simulink model "IEEE_39bus_load_increase_vol1"  (R2024b)
settings: Solver=ode23tb  StartTime=0.0  StopTime=500  MaxStep=1/60  RelTol=1e-2  AbsTol=1e-1  EnableMultiTasking=on
PreLoadFcn:
  | NE39bus_data;
  | PSSMODEL=1;
  | LPSS=0;
  | WAPSS=0;
  | WAPSS2=0;
values from neighbouring files (symbols this model uses):
  deg = [19.62;0;2.466;4.423;3.398;5.698;8.494;2.181;7.784;-3.646]*pi/180    [main_39.m]
  ki_sapc = 0.02*2.5/4    (= 0.0125)    [main_39.m]
  kp = 5*ones(10,1)    [main_39.m]
  kp_sapc = 0.15*1.25    (= 0.1875)    [main_39.m]
  line = [     1	2	0.0035	0.0411	0.6987	0	100	345 ... (first row only)    [main_39.m]
  P_base = mac_con(:,3).*[0.5609;0.6011;0.6995;0.6432;0.5143;0.6634;0.5676;0.5897;0.8444;0.3464]    [main_39.m]
  P_cmd = [1.140 	1.060 	1.100 	1.120 	0	1.060 	1.115 	1.160 	1.175 	1.000 ]    [main_39.m]
  Pmax = [1.20; 1.10; 1.15; 1.15;1.10;1.10;1.15;1.20;1.20;1.00]    [main_39.m]
  Pmin = 2-Pmax    [main_39.m]
  s = 10    [main_39.m]
  ts_pi = 5    [main_39.m]
  Udc = 2*Bus(mac_con(:,2),2)*1e3    [main_39.m]
  V_m = [1.03;0.982;0.9831;0.9972;1.0123;1.0493;1.0635;1.0278;1.0265;1.048]*sqrt(2/3)    [main_39.m]
undefined symbols (not defined in the file or in its folder): D1, Delta
libraries: spsThreePhaseVIMeasurementLib x40, spsThreePhasePISectionLineLib x34, spsThreePhaseParallelRLCLoadLib x21, spsThreePhaseTransformerTwoWindingsLib x13, spsMeanLib x12, slpidlib x12, spsLoadFlowBusLib x10, spsPLL3phLib x10, spsPowerPositiveSequenceLib x10, spsDCVoltageSourceLib x10, simulink x10, spsUniversalBridgeLib x10
(part 3 of 4)

== system IEEE_39bus_load_increase_vol1/VSC3/sapc ==
  In1 : Inport
  In2 : Inport  Port=2
  Abs1 : Abs  SaturateOnIntegerOverflow=off
  Constant : Constant  Value=kp_sapc
  Constant1 : Constant  Value=ki_sapc
  Constant2 : Constant  Value=1/0.015
  Constant3 : Constant  Value=1.5
  Constant4 : Constant  Value=0.016
  Delay : Delay  DelayLength=1  InitialCondition=0  SampleTime=1e-4
  Delay1 : Delay  DelayLength=1  InitialCondition=0  SampleTime=1e-4
  Delay2 : Delay  DelayLength=1  InitialCondition=0  SampleTime=1e-4
  Discrete PID Controller : slpidlib/PID Controller  Controller=PI  Form=Parallel  TimeDomain=Discrete-time  UseExternalTs=off  SampleTime=-1  IntegratorMethod=Forward Euler  FilterMethod=Forward Euler  ControllerParametersSource=external  P=kp_sapc  I=ki_sapc  UseKiTs=off  D=0  UseExternalDerivativeSource=off  N=100  UseFilter=on  TunerSelectOption=Transfer Function Based (PID Tuner App)  InitialConditionSource=internal  InitialConditionForIntegrator=0  InitialConditionForFilter=0  DifferentiatorICPrevScaledInput=0  ExternalReset=none  TrackingMode=off  Kt=1  LimitOutput=off  SatLimitsSource=internal  UpperSaturationLimit=inf  LowerSaturationLimit=-inf  LinearizeAsGain=off  AntiWindupMode=none  Kb=1  LimitIntegrator=off  UpperIntegratorSaturationLimit=inf  LowerIntegratorSaturationLimit=-inf  POutMin=[]  POutMax=[]  IOutMin=[]  IOutMax=[]  DOutMin=[]  DOutMax=[]  NOutMin=[]  NOutMax=[]  SumOutMin=[]  SumOutMax=[]  SaturationOutMin=[]  SaturationOutMax=[]  PParamMin=[]  PParamMax=[]  IParamMin=[]  IParamMax=[]  DParamMin=[]  DParamMax=[]  NParamMin=[]  NParamMax=[]  KbParamMin=[]  KbParamMax=[]  KtParamMin=[]  KtParamMax=[]  KbOutMin=[]  KbOutMax=[]  KtOutMin=[]  KtOutMax=[]  IntegratorOutMin=[]  IntegratorOutMax=[]  FilterOutMin=[]  FilterOutMax=[]  SumI1OutMin=[]  SumI1OutMax=[]  SumI2OutMin=[]  SumI2OutMax=[]  SumI3OutMin=[]  SumI3OutMax=[]  SumI4OutMin=[]  SumI4OutMax=[]  SumDOutMin=[]  SumDOutMax=[]  DifferentiatorOutMin=[]  DifferentiatorOutMax=[]  FilterDiffOutCoefMin=[]  FilterDiffOutCoefMax=[]  ReciprocalOutMin=[]  ReciprocalOutMax=[]  SumDenOutMin=[]  SumDenOutMax=[]  SumNumOutMin=[]  SumNumOutMax=[]  DivideOutMin=[]  DivideOutMax=[]  UdiffTsProdOutMin=[]  UdiffTsProdOutMax=[]  NTsProdOutMin=[]  NTsProdOutMax=[]  UintegralTsProdOutMin=[]  UintegralTsProdOutMax=[]  UngainTsProdOutMin=[]  UngainTsProdOutMax=[]  ClampingZeroOutDataTypeStr=Inherit: Inherit via back propagation  ClampingZeroOutMin=[]  ClampingZeroOutMax=[]  FilterDenConstantOutDataTypeStr=Inherit: Inherit via back propagation  FilterDenConstantOutMin=[]  FilterDenConstantOutMax=[]  PCopyOutDataTypeStr=Inherit: Inherit via back propagation  PCopyOutMin=[]  PCopyOutMax=[]  NCopyOutDataTypeStr=Inherit: Inherit via back propagation  NCopyOutMin=[]  NCopyOutMax=[]  IntegratorContinuousStateAttributes=''  IntegratorStateMustResolveToSignalObject=off  IntegratorRTWStateStorageClass=Auto  FilterContinuousStateAttributes=''  FilterStateMustResolveToSignalObject=off  FilterRTWStateStorageClass=Auto  ParallelPVariant=ExternalParameters  IdealPVariant=Disabled  IVariant=ExternalParameters  DVariant=Disabled  IntegratorVariant=Discrete  SatVariant=Disabled  AWVariant=Passthrough  PCopyVariant=Disabled  TRVariant=Disabled  FdbkBlocksVariant=Forward  IdealPFdbkVariant=Disabled  SatFdbkVariant=Disabled  DerivativeFilterVariant=Disabled  NVariant=Disabled  NCopyVariant=Disabled_SignalSpec  FilterICVariant=Disabled  IntegratorICVariant=InternalICs  ExternalResetVariant=Disabled  TRSumVariant=Passthrough  SumFdbkVariant=Disabled  SumVariant=Sum_PI  TsampFilterVariant=InternalTs  TsampNgainVariant=Passthrough  TsampIntegralVariant=Disabled_SignalSpec  ExternalSaturationOutDataTypeStr=Inherit: Same as second input  DerivativeSourceVariant=Disabled  PreIntVariant=InternalPreInt
      settings: LibrarySourceBlock=simulink/Discrete/Discrete PID Controller
  Gain1 : Gain  Gain=1/0.015/0.015
  Gain2 : Gain  Gain=1/2
  Gain4 : Gain  Gain=P_base(3)/1e3
  Product{,1..5} (6 alike) : Product
  Saturation : Saturate  UpperLimit=1  LowerLimit=1
  Saturation1 : Saturate  UpperLimit=1  LowerLimit=0
  Scope1 : Scope  NumInputPorts=3
  Scope2 : Scope  NumInputPorts=2
  Step : Step  Time=15  SampleTime=0
  Sum : Sum  Inputs=|+-
  Sum1 : Sum  Inputs=|+-
  Sum2 : Sum  Inputs=|+-
  Sum3 : Sum  Inputs=|++
  Zero-Order Hold : ZeroOrderHold  SampleTime=ts_pi
  delta : Outport
  tag scope: delta_sapc3=global
  wires:
  Product/1 -> [delta_sapc3], Scope1/3, Discrete PID Controller/1
  Step/1 -> Product/2
  Sum/1 -> Gain4/1
  Discrete PID Controller/1 -> Scope1/1, Zero-Order Hold/1
  In1/1 -> Sum/1
  In2/1 -> Sum/2
  Zero-Order Hold/1 -> Scope1/2, Delay1/1
  Product2/1 -> Scope2/2, Discrete PID Controller/3
  Constant/1 -> Product1/1
  Saturation/1 -> Product2/1, Product1/2
  Product1/1 -> Scope2/1, Discrete PID Controller/2
  Constant1/1 -> Product2/2
  Constant4/1 -> Sum1/1
  Abs1/1 -> Product5/2, Sum1/2
  Constant3/1 -> Sum2/1
  Product3/1 -> Gain1/1
  Gain1/1 -> Delay/1
  Sum1/1 -> Product3/1, Product3/2
  Gain4/1 -> Abs1/1, Product/1
  Delay/1 -> Sum2/2
  Delay1/1 -> delta/1
  Product5/1 -> Saturation1/1
  Saturation1/1 -> Product4/1
  Constant2/1 -> Product5/1
  Sum2/1 -> Product4/2
  Product4/1 -> Sum3/2, Delay2/1
  Delay2/1 -> Sum3/1
  Gain2/1 -> Saturation/1
  Sum3/1 -> Gain2/1

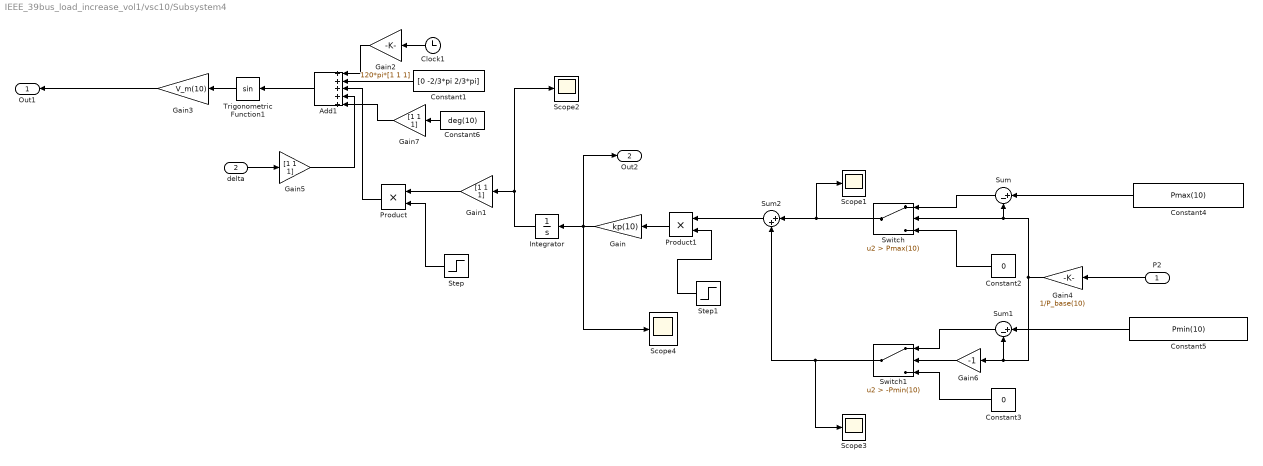
== system IEEE_39bus_load_increase_vol1/vsc10/Subsystem4 ==
  P2 : Inport
  delta : Inport  Port=2
  Add1 : Sum  Inputs=+++++
  Clock1 : Clock
  Constant1 : Constant  Value="[0  -2/3*pi   2/3*pi]"
  Constant2 : Constant  Value=0
  Constant3 : Constant  Value=0
  Constant4 : Constant  Value=Pmax(10)
  Constant5 : Constant  Value=Pmin(10)
  Constant6 : Constant  Value=deg(10)
  Gain : Gain  Gain=kp(10)
  Gain1 : Gain  Gain=[1 1 1]
  Gain2 : Gain  Gain=120*pi*[1 1 1]
  Gain3 : Gain  Gain=V_m(10)
  Gain4 : Gain  Gain=1/P_base(10)
  Gain5 : Gain  Gain=[1 1 1]
  Gain6 : Gain  Gain=-1
  Gain7 : Gain  Gain=[1 1 1]
  Integrator : Integrator
  Product : Product
  Product1 : Product
  Scope{1..4} (4 alike) : Scope
  Step : Step  Time=5  SampleTime=0
  Step1 : Step  Time=5  SampleTime=0
  Sum : Sum  Inputs=|+-
  Sum1 : Sum  Inputs=|+-
  Sum2 : Sum  Inputs=|++
  Switch : Switch  Criteria=u2 > Threshold  Threshold=Pmax(10)  SaturateOnIntegerOverflow=off  InputSameDT=off
  Switch1 : Switch  Criteria=u2 > Threshold  Threshold=-Pmin(10)  SaturateOnIntegerOverflow=off  InputSameDT=off
  Trigonometric Function1 : Trigonometry
  Out1 : Outport
  Out2 : Outport  Port=2
  wires:
  Clock1/1 -> Gain2/1
  Constant1/1 -> Add1/2
  Gain2/1 -> Add1/1
  Add1/1 -> Trigonometric Function1/1
  Gain1/1 -> Product/1
  Step/1 -> Product/2
  Product/1 -> Add1/3
  Trigonometric Function1/1 -> Gain3/1
  Gain3/1 -> Out1/1
  Gain/1 -> Out2/1, Scope4/1, Integrator/1
  P2/1 -> Gain4/1
  delta/1 -> Gain5/1
  Gain5/1 -> Add1/4
  Step1/1 -> Product1/2
  Product1/1 -> Gain/1
  Constant4/1 -> Sum/1
  Sum/1 -> Switch/1
  Constant2/1 -> Switch/3
  Constant5/1 -> Sum1/1
  Sum1/1 -> Switch1/1
  Gain4/1 -> Gain6/1, Sum1/2, Sum/2, Switch/2
  Constant3/1 -> Switch1/3
  Gain6/1 -> Switch1/2
  Switch/1 -> Scope1/1, Sum2/1
  Switch1/1 -> Scope3/1, Sum2/2
  Sum2/1 -> Product1/1
  Constant6/1 -> Gain7/1
  Gain7/1 -> Add1/5
  Integrator/1 -> Scope2/1, Gain1/1

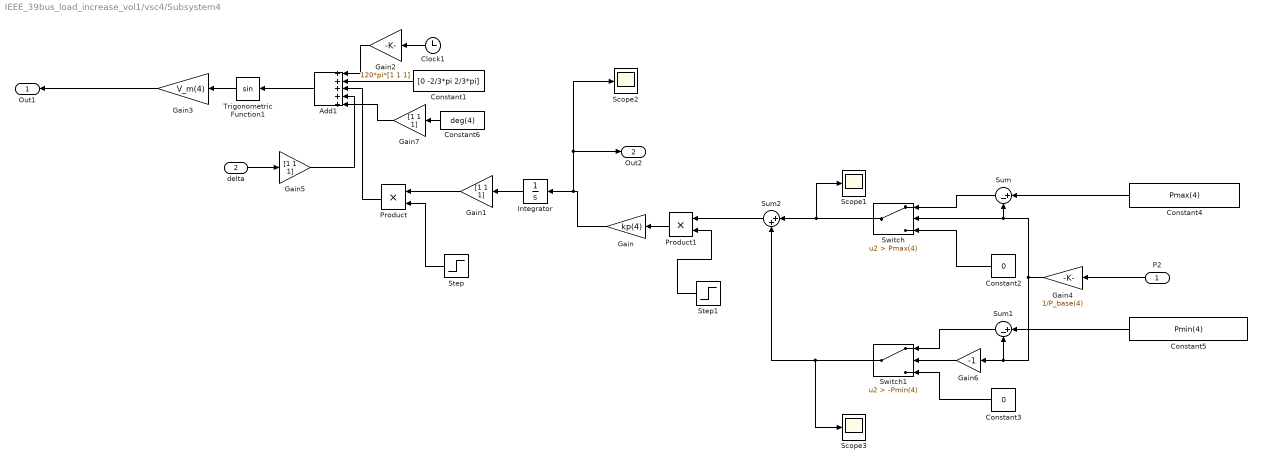
== system IEEE_39bus_load_increase_vol1/vsc4/Subsystem4 ==
  P2 : Inport
  delta : Inport  Port=2
  Add1 : Sum  Inputs=+++++
  Clock1 : Clock
  Constant1 : Constant  Value="[0  -2/3*pi   2/3*pi]"
  Constant2 : Constant  Value=0
  Constant3 : Constant  Value=0
  Constant4 : Constant  Value=Pmax(4)
  Constant5 : Constant  Value=Pmin(4)
  Constant6 : Constant  Value=deg(4)
  Gain : Gain  Gain=kp(4)
  Gain1 : Gain  Gain=[1 1 1]
  Gain2 : Gain  Gain=120*pi*[1 1 1]
  Gain3 : Gain  Gain=V_m(4)
  Gain4 : Gain  Gain=1/P_base(4)
  Gain5 : Gain  Gain=[1 1 1]
  Gain6 : Gain  Gain=-1
  Gain7 : Gain  Gain=[1 1 1]
  Integrator : Integrator
  Product : Product
  Product1 : Product
  Scope1 : Scope
  Scope2 : Scope
  Scope3 : Scope
  Step : Step  Time=5  SampleTime=0
  Step1 : Step  Time=5  SampleTime=0
  Sum : Sum  Inputs=|+-
  Sum1 : Sum  Inputs=|+-
  Sum2 : Sum  Inputs=|++
  Switch : Switch  Criteria=u2 > Threshold  Threshold=Pmax(4)  SaturateOnIntegerOverflow=off  InputSameDT=off
  Switch1 : Switch  Criteria=u2 > Threshold  Threshold=-Pmin(4)  SaturateOnIntegerOverflow=off  InputSameDT=off
  Trigonometric Function1 : Trigonometry
  Out1 : Outport
  Out2 : Outport  Port=2
  wires:
  Clock1/1 -> Gain2/1
  Constant1/1 -> Add1/2
  Gain2/1 -> Add1/1
  Add1/1 -> Trigonometric Function1/1
  Gain1/1 -> Product/1
  Step/1 -> Product/2
  Product/1 -> Add1/3
  Trigonometric Function1/1 -> Gain3/1
  Gain3/1 -> Out1/1
  P2/1 -> Gain4/1
  delta/1 -> Gain5/1
  Gain5/1 -> Add1/4
  Step1/1 -> Product1/2
  Constant4/1 -> Sum/1
  Sum/1 -> Switch/1
  Constant2/1 -> Switch/3
  Constant5/1 -> Sum1/1
  Sum1/1 -> Switch1/1
  Gain4/1 -> Gain6/1, Sum1/2, Sum/2, Switch/2
  Constant3/1 -> Switch1/3
  Gain6/1 -> Switch1/2
  Switch/1 -> Scope1/1, Sum2/1
  Switch1/1 -> Scope3/1, Sum2/2
  Sum2/1 -> Product1/1
  Constant6/1 -> Gain7/1
  Gain7/1 -> Add1/5
  Product1/1 -> Gain/1
  Integrator/1 -> Gain1/1
  Gain/1 -> Out2/1, Scope2/1, Integrator/1

== system IEEE_39bus_load_increase_vol1/vsc4/sapc ==
  In1 : Inport
  In2 : Inport  Port=2
  Discrete PID Controller : slpidlib/PID Controller  Controller=PI  Form=Parallel  TimeDomain=Discrete-time  UseExternalTs=off  SampleTime=-1  IntegratorMethod=Forward Euler  FilterMethod=Forward Euler  ControllerParametersSource=internal  P=kp_sapc*0.5  I=ki_sapc*0.5  UseKiTs=off  D=0  UseExternalDerivativeSource=off  N=100  UseFilter=on  TunerSelectOption=Transfer Function Based (PID Tuner App)  InitialConditionSource=internal  InitialConditionForIntegrator=0  InitialConditionForFilter=0  DifferentiatorICPrevScaledInput=0  ExternalReset=none  TrackingMode=off  Kt=1  LimitOutput=off  SatLimitsSource=internal  UpperSaturationLimit=inf  LowerSaturationLimit=-inf  LinearizeAsGain=off  AntiWindupMode=none  Kb=1  LimitIntegrator=off  UpperIntegratorSaturationLimit=inf  LowerIntegratorSaturationLimit=-inf  POutMin=[]  POutMax=[]  IOutMin=[]  IOutMax=[]  DOutMin=[]  DOutMax=[]  NOutMin=[]  NOutMax=[]  SumOutMin=[]  SumOutMax=[]  SaturationOutMin=[]  SaturationOutMax=[]  PParamMin=[]  PParamMax=[]  IParamMin=[]  IParamMax=[]  DParamMin=[]  DParamMax=[]  NParamMin=[]  NParamMax=[]  KbParamMin=[]  KbParamMax=[]  KtParamMin=[]  KtParamMax=[]  KbOutMin=[]  KbOutMax=[]  KtOutMin=[]  KtOutMax=[]  IntegratorOutMin=[]  IntegratorOutMax=[]  FilterOutMin=[]  FilterOutMax=[]  SumI1OutMin=[]  SumI1OutMax=[]  SumI2OutMin=[]  SumI2OutMax=[]  SumI3OutMin=[]  SumI3OutMax=[]  SumI4OutMin=[]  SumI4OutMax=[]  SumDOutMin=[]  SumDOutMax=[]  DifferentiatorOutMin=[]  DifferentiatorOutMax=[]  FilterDiffOutCoefMin=[]  FilterDiffOutCoefMax=[]  ReciprocalOutMin=[]  ReciprocalOutMax=[]  SumDenOutMin=[]  SumDenOutMax=[]  SumNumOutMin=[]  SumNumOutMax=[]  DivideOutMin=[]  DivideOutMax=[]  UdiffTsProdOutMin=[]  UdiffTsProdOutMax=[]  NTsProdOutMin=[]  NTsProdOutMax=[]  UintegralTsProdOutMin=[]  UintegralTsProdOutMax=[]  UngainTsProdOutMin=[]  UngainTsProdOutMax=[]  ClampingZeroOutDataTypeStr=Inherit: Inherit via back propagation  ClampingZeroOutMin=[]  ClampingZeroOutMax=[]  FilterDenConstantOutDataTypeStr=Inherit: Inherit via back propagation  FilterDenConstantOutMin=[]  FilterDenConstantOutMax=[]  PCopyOutDataTypeStr=Inherit: Inherit via back propagation  PCopyOutMin=[]  PCopyOutMax=[]  NCopyOutDataTypeStr=Inherit: Inherit via back propagation  NCopyOutMin=[]  NCopyOutMax=[]  IntegratorContinuousStateAttributes=''  IntegratorStateMustResolveToSignalObject=off  IntegratorRTWStateStorageClass=Auto  FilterContinuousStateAttributes=''  FilterStateMustResolveToSignalObject=off  FilterRTWStateStorageClass=Auto  ParallelPVariant=InternalParameters  IdealPVariant=Disabled  IVariant=InternalParameters  DVariant=Disabled  IntegratorVariant=Discrete  SatVariant=Disabled  AWVariant=Passthrough  PCopyVariant=Disabled  TRVariant=Disabled  FdbkBlocksVariant=Forward  IdealPFdbkVariant=Disabled  SatFdbkVariant=Disabled  DerivativeFilterVariant=Disabled  NVariant=Disabled  NCopyVariant=Disabled_SignalSpec  FilterICVariant=Disabled  IntegratorICVariant=InternalICs  ExternalResetVariant=Disabled  TRSumVariant=Passthrough  SumFdbkVariant=Disabled  SumVariant=Sum_PI  TsampFilterVariant=InternalTs  TsampNgainVariant=Passthrough  TsampIntegralVariant=Disabled_SignalSpec  ExternalSaturationOutDataTypeStr=Inherit: Same as second input  DerivativeSourceVariant=Disabled  PreIntVariant=InternalPreInt
      settings: LibrarySourceBlock=simulink/Discrete/Discrete PID Controller
  Gain4 : Gain  Gain=P_base(4)/1e3
  Product : Product
  Scope1 : Scope  NumInputPorts=2
  Step : Step  Time=15  SampleTime=0
  Sum : Sum  Inputs=|+-
  Zero-Order Hold : ZeroOrderHold  SampleTime=ts_pi
  delta : Outport
  tag scope: delta_sapc4=global
  wires:
  Product/1 -> [delta_sapc4], Scope1/2, Discrete PID Controller/1
  Step/1 -> Product/2
  Sum/1 -> Gain4/1
  Discrete PID Controller/1 -> Zero-Order Hold/1, Scope1/1
  In1/1 -> Sum/1
  In2/1 -> Sum/2
  Zero-Order Hold/1 -> delta/1
  Gain4/1 -> Product/1

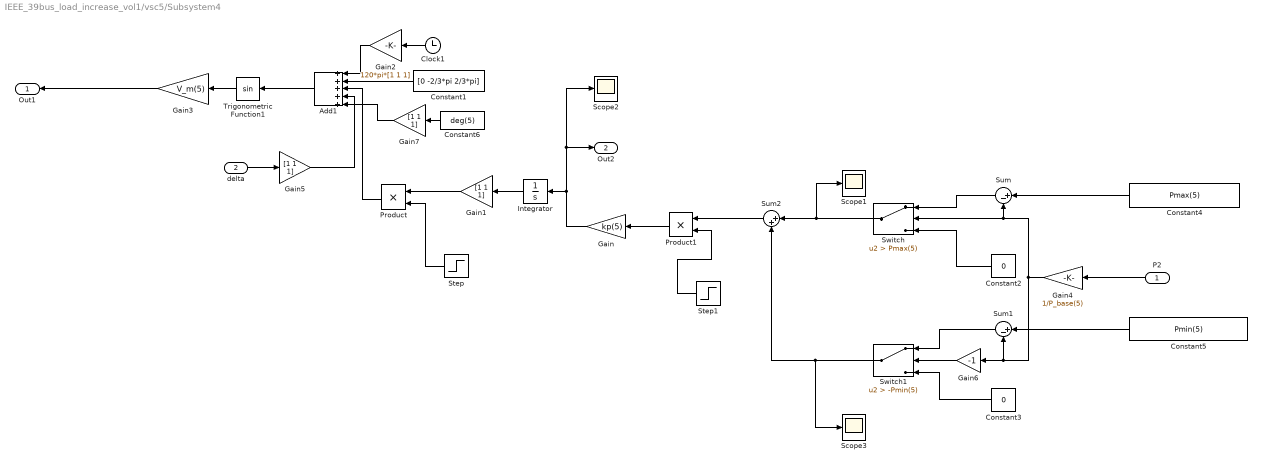
== system IEEE_39bus_load_increase_vol1/vsc5/Subsystem4 ==
  P2 : Inport
  delta : Inport  Port=2
  Add1 : Sum  Inputs=+++++
  Clock1 : Clock
  Constant1 : Constant  Value="[0  -2/3*pi   2/3*pi]"
  Constant2 : Constant  Value=0
  Constant3 : Constant  Value=0
  Constant4 : Constant  Value=Pmax(5)
  Constant5 : Constant  Value=Pmin(5)
  Constant6 : Constant  Value=deg(5)
  Gain : Gain  Gain=kp(5)
  Gain1 : Gain  Gain=[1 1 1]
  Gain2 : Gain  Gain=120*pi*[1 1 1]
  Gain3 : Gain  Gain=V_m(5)
  Gain4 : Gain  Gain=1/P_base(5)
  Gain5 : Gain  Gain=[1 1 1]
  Gain6 : Gain  Gain=-1
  Gain7 : Gain  Gain=[1 1 1]
  Integrator : Integrator
  Product : Product
  Product1 : Product
  Scope1 : Scope
  Scope2 : Scope
  Scope3 : Scope
  Step : Step  Time=5  SampleTime=0
  Step1 : Step  Time=5  SampleTime=0
  Sum : Sum  Inputs=|+-
  Sum1 : Sum  Inputs=|+-
  Sum2 : Sum  Inputs=|++
  Switch : Switch  Criteria=u2 > Threshold  Threshold=Pmax(5)  SaturateOnIntegerOverflow=off  InputSameDT=off
  Switch1 : Switch  Criteria=u2 > Threshold  Threshold=-Pmin(5)  SaturateOnIntegerOverflow=off  InputSameDT=off
  Trigonometric Function1 : Trigonometry
  Out1 : Outport
  Out2 : Outport  Port=2
  wires:
  Clock1/1 -> Gain2/1
  Constant1/1 -> Add1/2
  Gain2/1 -> Add1/1
  Add1/1 -> Trigonometric Function1/1
  Gain1/1 -> Product/1
  Step/1 -> Product/2
  Product/1 -> Add1/3
  Trigonometric Function1/1 -> Gain3/1
  Gain3/1 -> Out1/1
  P2/1 -> Gain4/1
  delta/1 -> Gain5/1
  Gain5/1 -> Add1/4
  Step1/1 -> Product1/2
  Constant4/1 -> Sum/1
  Sum/1 -> Switch/1
  Constant2/1 -> Switch/3
  Constant5/1 -> Sum1/1
  Sum1/1 -> Switch1/1
  Gain4/1 -> Gain6/1, Sum1/2, Sum/2, Switch/2
  Constant3/1 -> Switch1/3
  Gain6/1 -> Switch1/2
  Switch/1 -> Scope1/1, Sum2/1
  Switch1/1 -> Scope3/1, Sum2/2
  Sum2/1 -> Product1/1
  Constant6/1 -> Gain7/1
  Gain7/1 -> Add1/5
  Integrator/1 -> Gain1/1
  Gain/1 -> Integrator/1, Scope2/1, Out2/1
  Product1/1 -> Gain/1

== system IEEE_39bus_load_increase_vol1/vsc5/sapc ==
  In1 : Inport
  In2 : Inport  Port=2
  Discrete PID Controller : slpidlib/PID Controller  Controller=PI  Form=Parallel  TimeDomain=Discrete-time  UseExternalTs=off  SampleTime=-1  IntegratorMethod=Forward Euler  FilterMethod=Forward Euler  ControllerParametersSource=internal  P=kp_sapc  I=ki_sapc  UseKiTs=off  D=0  UseExternalDerivativeSource=off  N=100  UseFilter=on  TunerSelectOption=Transfer Function Based (PID Tuner App)  InitialConditionSource=internal  InitialConditionForIntegrator=0  InitialConditionForFilter=0  DifferentiatorICPrevScaledInput=0  ExternalReset=none  TrackingMode=off  Kt=1  LimitOutput=off  SatLimitsSource=internal  UpperSaturationLimit=inf  LowerSaturationLimit=-inf  LinearizeAsGain=off  AntiWindupMode=none  Kb=1  LimitIntegrator=off  UpperIntegratorSaturationLimit=inf  LowerIntegratorSaturationLimit=-inf  POutMin=[]  POutMax=[]  IOutMin=[]  IOutMax=[]  DOutMin=[]  DOutMax=[]  NOutMin=[]  NOutMax=[]  SumOutMin=[]  SumOutMax=[]  SaturationOutMin=[]  SaturationOutMax=[]  PParamMin=[]  PParamMax=[]  IParamMin=[]  IParamMax=[]  DParamMin=[]  DParamMax=[]  NParamMin=[]  NParamMax=[]  KbParamMin=[]  KbParamMax=[]  KtParamMin=[]  KtParamMax=[]  KbOutMin=[]  KbOutMax=[]  KtOutMin=[]  KtOutMax=[]  IntegratorOutMin=[]  IntegratorOutMax=[]  FilterOutMin=[]  FilterOutMax=[]  SumI1OutMin=[]  SumI1OutMax=[]  SumI2OutMin=[]  SumI2OutMax=[]  SumI3OutMin=[]  SumI3OutMax=[]  SumI4OutMin=[]  SumI4OutMax=[]  SumDOutMin=[]  SumDOutMax=[]  DifferentiatorOutMin=[]  DifferentiatorOutMax=[]  FilterDiffOutCoefMin=[]  FilterDiffOutCoefMax=[]  ReciprocalOutMin=[]  ReciprocalOutMax=[]  SumDenOutMin=[]  SumDenOutMax=[]  SumNumOutMin=[]  SumNumOutMax=[]  DivideOutMin=[]  DivideOutMax=[]  UdiffTsProdOutMin=[]  UdiffTsProdOutMax=[]  NTsProdOutMin=[]  NTsProdOutMax=[]  UintegralTsProdOutMin=[]  UintegralTsProdOutMax=[]  UngainTsProdOutMin=[]  UngainTsProdOutMax=[]  ClampingZeroOutDataTypeStr=Inherit: Inherit via back propagation  ClampingZeroOutMin=[]  ClampingZeroOutMax=[]  FilterDenConstantOutDataTypeStr=Inherit: Inherit via back propagation  FilterDenConstantOutMin=[]  FilterDenConstantOutMax=[]  PCopyOutDataTypeStr=Inherit: Inherit via back propagation  PCopyOutMin=[]  PCopyOutMax=[]  NCopyOutDataTypeStr=Inherit: Inherit via back propagation  NCopyOutMin=[]  NCopyOutMax=[]  IntegratorContinuousStateAttributes=''  IntegratorStateMustResolveToSignalObject=off  IntegratorRTWStateStorageClass=Auto  FilterContinuousStateAttributes=''  FilterStateMustResolveToSignalObject=off  FilterRTWStateStorageClass=Auto  ParallelPVariant=InternalParameters  IdealPVariant=Disabled  IVariant=InternalParameters  DVariant=Disabled  IntegratorVariant=Discrete  SatVariant=Disabled  AWVariant=Passthrough  PCopyVariant=Disabled  TRVariant=Disabled  FdbkBlocksVariant=Forward  IdealPFdbkVariant=Disabled  SatFdbkVariant=Disabled  DerivativeFilterVariant=Disabled  NVariant=Disabled  NCopyVariant=Disabled_SignalSpec  FilterICVariant=Disabled  IntegratorICVariant=InternalICs  ExternalResetVariant=Disabled  TRSumVariant=Passthrough  SumFdbkVariant=Disabled  SumVariant=Sum_PI  TsampFilterVariant=InternalTs  TsampNgainVariant=Passthrough  TsampIntegralVariant=Disabled_SignalSpec  ExternalSaturationOutDataTypeStr=Inherit: Same as second input  DerivativeSourceVariant=Disabled  PreIntVariant=InternalPreInt
      settings: LibrarySourceBlock=simulink/Discrete/Discrete PID Controller
  Gain4 : Gain  Gain=P_base(5)/1e3
  Product : Product
  Scope1 : Scope  NumInputPorts=2
  Step : Step  Time=15  SampleTime=0
  Sum : Sum  Inputs=|+-
  Zero-Order Hold : ZeroOrderHold  SampleTime=ts_pi
  delta : Outport
  tag scope: delta_sapc5=global
  wires:
  Product/1 -> [delta_sapc5], Scope1/2, Discrete PID Controller/1
  Step/1 -> Product/2
  Sum/1 -> Gain4/1
  Discrete PID Controller/1 -> Zero-Order Hold/1, Scope1/1
  In1/1 -> Sum/1
  In2/1 -> Sum/2
  Zero-Order Hold/1 -> delta/1
  Gain4/1 -> Product/1

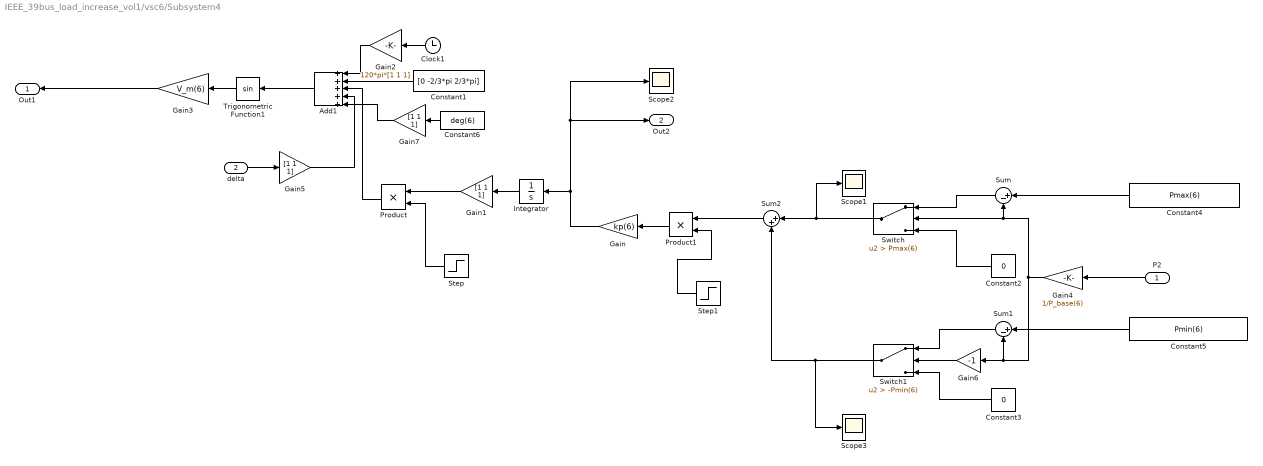
== system IEEE_39bus_load_increase_vol1/vsc6/Subsystem4 ==
  P2 : Inport
  delta : Inport  Port=2
  Add1 : Sum  Inputs=+++++
  Clock1 : Clock
  Constant1 : Constant  Value="[0  -2/3*pi   2/3*pi]"
  Constant2 : Constant  Value=0
  Constant3 : Constant  Value=0
  Constant4 : Constant  Value=Pmax(6)
  Constant5 : Constant  Value=Pmin(6)
  Constant6 : Constant  Value=deg(6)
  Gain : Gain  Gain=kp(6)
  Gain1 : Gain  Gain=[1 1 1]
  Gain2 : Gain  Gain=120*pi*[1 1 1]
  Gain3 : Gain  Gain=V_m(6)
  Gain4 : Gain  Gain=1/P_base(6)
  Gain5 : Gain  Gain=[1 1 1]
  Gain6 : Gain  Gain=-1
  Gain7 : Gain  Gain=[1 1 1]
  Integrator : Integrator
  Product : Product
  Product1 : Product
  Scope1 : Scope
  Scope2 : Scope
  Scope3 : Scope
  Step : Step  Time=5  SampleTime=0
  Step1 : Step  Time=5  SampleTime=0
  Sum : Sum  Inputs=|+-
  Sum1 : Sum  Inputs=|+-
  Sum2 : Sum  Inputs=|++
  Switch : Switch  Criteria=u2 > Threshold  Threshold=Pmax(6)  SaturateOnIntegerOverflow=off  InputSameDT=off
  Switch1 : Switch  Criteria=u2 > Threshold  Threshold=-Pmin(6)  SaturateOnIntegerOverflow=off  InputSameDT=off
  Trigonometric Function1 : Trigonometry
  Out1 : Outport
  Out2 : Outport  Port=2
  wires:
  Clock1/1 -> Gain2/1
  Constant1/1 -> Add1/2
  Gain2/1 -> Add1/1
  Add1/1 -> Trigonometric Function1/1
  Gain1/1 -> Product/1
  Step/1 -> Product/2
  Product/1 -> Add1/3
  Trigonometric Function1/1 -> Gain3/1
  Gain3/1 -> Out1/1
  P2/1 -> Gain4/1
  delta/1 -> Gain5/1
  Gain5/1 -> Add1/4
  Step1/1 -> Product1/2
  Constant4/1 -> Sum/1
  Sum/1 -> Switch/1
  Constant2/1 -> Switch/3
  Constant5/1 -> Sum1/1
  Sum1/1 -> Switch1/1
  Gain4/1 -> Gain6/1, Sum1/2, Sum/2, Switch/2
  Constant3/1 -> Switch1/3
  Gain6/1 -> Switch1/2
  Switch/1 -> Scope1/1, Sum2/1
  Switch1/1 -> Scope3/1, Sum2/2
  Sum2/1 -> Product1/1
  Constant6/1 -> Gain7/1
  Gain7/1 -> Add1/5
  Product1/1 -> Gain/1
  Integrator/1 -> Gain1/1
  Gain/1 -> Scope2/1, Out2/1, Integrator/1

== system IEEE_39bus_load_increase_vol1/vsc6/sapc ==
  In1 : Inport
  In2 : Inport  Port=2
  Discrete PID Controller : slpidlib/PID Controller  Controller=PI  Form=Parallel  TimeDomain=Discrete-time  UseExternalTs=off  SampleTime=-1  IntegratorMethod=Forward Euler  FilterMethod=Forward Euler  ControllerParametersSource=internal  P=kp_sapc  I=ki_sapc  UseKiTs=off  D=0  UseExternalDerivativeSource=off  N=100  UseFilter=on  TunerSelectOption=Transfer Function Based (PID Tuner App)  InitialConditionSource=internal  InitialConditionForIntegrator=0  InitialConditionForFilter=0  DifferentiatorICPrevScaledInput=0  ExternalReset=none  TrackingMode=off  Kt=1  LimitOutput=off  SatLimitsSource=internal  UpperSaturationLimit=inf  LowerSaturationLimit=-inf  LinearizeAsGain=off  AntiWindupMode=none  Kb=1  LimitIntegrator=off  UpperIntegratorSaturationLimit=inf  LowerIntegratorSaturationLimit=-inf  POutMin=[]  POutMax=[]  IOutMin=[]  IOutMax=[]  DOutMin=[]  DOutMax=[]  NOutMin=[]  NOutMax=[]  SumOutMin=[]  SumOutMax=[]  SaturationOutMin=[]  SaturationOutMax=[]  PParamMin=[]  PParamMax=[]  IParamMin=[]  IParamMax=[]  DParamMin=[]  DParamMax=[]  NParamMin=[]  NParamMax=[]  KbParamMin=[]  KbParamMax=[]  KtParamMin=[]  KtParamMax=[]  KbOutMin=[]  KbOutMax=[]  KtOutMin=[]  KtOutMax=[]  IntegratorOutMin=[]  IntegratorOutMax=[]  FilterOutMin=[]  FilterOutMax=[]  SumI1OutMin=[]  SumI1OutMax=[]  SumI2OutMin=[]  SumI2OutMax=[]  SumI3OutMin=[]  SumI3OutMax=[]  SumI4OutMin=[]  SumI4OutMax=[]  SumDOutMin=[]  SumDOutMax=[]  DifferentiatorOutMin=[]  DifferentiatorOutMax=[]  FilterDiffOutCoefMin=[]  FilterDiffOutCoefMax=[]  ReciprocalOutMin=[]  ReciprocalOutMax=[]  SumDenOutMin=[]  SumDenOutMax=[]  SumNumOutMin=[]  SumNumOutMax=[]  DivideOutMin=[]  DivideOutMax=[]  UdiffTsProdOutMin=[]  UdiffTsProdOutMax=[]  NTsProdOutMin=[]  NTsProdOutMax=[]  UintegralTsProdOutMin=[]  UintegralTsProdOutMax=[]  UngainTsProdOutMin=[]  UngainTsProdOutMax=[]  ClampingZeroOutDataTypeStr=Inherit: Inherit via back propagation  ClampingZeroOutMin=[]  ClampingZeroOutMax=[]  FilterDenConstantOutDataTypeStr=Inherit: Inherit via back propagation  FilterDenConstantOutMin=[]  FilterDenConstantOutMax=[]  PCopyOutDataTypeStr=Inherit: Inherit via back propagation  PCopyOutMin=[]  PCopyOutMax=[]  NCopyOutDataTypeStr=Inherit: Inherit via back propagation  NCopyOutMin=[]  NCopyOutMax=[]  IntegratorContinuousStateAttributes=''  IntegratorStateMustResolveToSignalObject=off  IntegratorRTWStateStorageClass=Auto  FilterContinuousStateAttributes=''  FilterStateMustResolveToSignalObject=off  FilterRTWStateStorageClass=Auto  ParallelPVariant=InternalParameters  IdealPVariant=Disabled  IVariant=InternalParameters  DVariant=Disabled  IntegratorVariant=Discrete  SatVariant=Disabled  AWVariant=Passthrough  PCopyVariant=Disabled  TRVariant=Disabled  FdbkBlocksVariant=Forward  IdealPFdbkVariant=Disabled  SatFdbkVariant=Disabled  DerivativeFilterVariant=Disabled  NVariant=Disabled  NCopyVariant=Disabled_SignalSpec  FilterICVariant=Disabled  IntegratorICVariant=InternalICs  ExternalResetVariant=Disabled  TRSumVariant=Passthrough  SumFdbkVariant=Disabled  SumVariant=Sum_PI  TsampFilterVariant=InternalTs  TsampNgainVariant=Passthrough  TsampIntegralVariant=Disabled_SignalSpec  ExternalSaturationOutDataTypeStr=Inherit: Same as second input  DerivativeSourceVariant=Disabled  PreIntVariant=InternalPreInt
      settings: LibrarySourceBlock=simulink/Discrete/Discrete PID Controller
  Gain4 : Gain  Gain=P_base(6)/1e3
  Goto10 : Goto  Commented=on  GotoTag=delta_sapc6  TagVisibility=global
  Product : Product
  Scope1 : Scope  NumInputPorts=2
  Step : Step  Time=15  SampleTime=0
  Sum : Sum  Inputs=|+-
  Zero-Order Hold : ZeroOrderHold  SampleTime=ts_pi
  delta : Outport
  wires:
  Product/1 -> Goto10/1, Scope1/2, Discrete PID Controller/1
  Step/1 -> Product/2
  Sum/1 -> Gain4/1
  Discrete PID Controller/1 -> Zero-Order Hold/1, Scope1/1
  In1/1 -> Sum/1
  In2/1 -> Sum/2
  Zero-Order Hold/1 -> delta/1
  Gain4/1 -> Product/1

== system IEEE_39bus_load_increase_vol1/vsc6/sapc1 ==
  In1 : Inport
  In2 : Inport  Port=2
  Abs1 : Abs  SaturateOnIntegerOverflow=off
  Constant : Constant  Value=kp_sapc
  Constant1 : Constant  Value=ki_sapc
  Constant2 : Constant  Value=1/0.015
  Constant3 : Constant
  Constant4 : Constant  Value=0.01
  Delay2 : Delay  DelayLength=1  InitialCondition=0  SampleTime=1e-4
  Discrete PID Controller : slpidlib/PID Controller  Controller=PI  Form=Parallel  TimeDomain=Discrete-time  UseExternalTs=off  SampleTime=-1  IntegratorMethod=Forward Euler  FilterMethod=Forward Euler  ControllerParametersSource=external  P=kp_sapc*2  I=ki_sapc*2  UseKiTs=off  D=0  UseExternalDerivativeSource=off  N=100  UseFilter=on  TunerSelectOption=Transfer Function Based (PID Tuner App)  InitialConditionSource=internal  InitialConditionForIntegrator=0  InitialConditionForFilter=0  DifferentiatorICPrevScaledInput=0  ExternalReset=none  TrackingMode=off  Kt=1  LimitOutput=off  SatLimitsSource=internal  UpperSaturationLimit=inf  LowerSaturationLimit=-inf  LinearizeAsGain=off  AntiWindupMode=none  Kb=1  LimitIntegrator=off  UpperIntegratorSaturationLimit=inf  LowerIntegratorSaturationLimit=-inf  POutMin=[]  POutMax=[]  IOutMin=[]  IOutMax=[]  DOutMin=[]  DOutMax=[]  NOutMin=[]  NOutMax=[]  SumOutMin=[]  SumOutMax=[]  SaturationOutMin=[]  SaturationOutMax=[]  PParamMin=[]  PParamMax=[]  IParamMin=[]  IParamMax=[]  DParamMin=[]  DParamMax=[]  NParamMin=[]  NParamMax=[]  KbParamMin=[]  KbParamMax=[]  KtParamMin=[]  KtParamMax=[]  KbOutMin=[]  KbOutMax=[]  KtOutMin=[]  KtOutMax=[]  IntegratorOutMin=[]  IntegratorOutMax=[]  FilterOutMin=[]  FilterOutMax=[]  SumI1OutMin=[]  SumI1OutMax=[]  SumI2OutMin=[]  SumI2OutMax=[]  SumI3OutMin=[]  SumI3OutMax=[]  SumI4OutMin=[]  SumI4OutMax=[]  SumDOutMin=[]  SumDOutMax=[]  DifferentiatorOutMin=[]  DifferentiatorOutMax=[]  FilterDiffOutCoefMin=[]  FilterDiffOutCoefMax=[]  ReciprocalOutMin=[]  ReciprocalOutMax=[]  SumDenOutMin=[]  SumDenOutMax=[]  SumNumOutMin=[]  SumNumOutMax=[]  DivideOutMin=[]  DivideOutMax=[]  UdiffTsProdOutMin=[]  UdiffTsProdOutMax=[]  NTsProdOutMin=[]  NTsProdOutMax=[]  UintegralTsProdOutMin=[]  UintegralTsProdOutMax=[]  UngainTsProdOutMin=[]  UngainTsProdOutMax=[]  ClampingZeroOutDataTypeStr=Inherit: Inherit via back propagation  ClampingZeroOutMin=[]  ClampingZeroOutMax=[]  FilterDenConstantOutDataTypeStr=Inherit: Inherit via back propagation  FilterDenConstantOutMin=[]  FilterDenConstantOutMax=[]  PCopyOutDataTypeStr=Inherit: Inherit via back propagation  PCopyOutMin=[]  PCopyOutMax=[]  NCopyOutDataTypeStr=Inherit: Inherit via back propagation  NCopyOutMin=[]  NCopyOutMax=[]  IntegratorContinuousStateAttributes=''  IntegratorStateMustResolveToSignalObject=off  IntegratorRTWStateStorageClass=Auto  FilterContinuousStateAttributes=''  FilterStateMustResolveToSignalObject=off  FilterRTWStateStorageClass=Auto  ParallelPVariant=ExternalParameters  IdealPVariant=Disabled  IVariant=ExternalParameters  DVariant=Disabled  IntegratorVariant=Discrete  SatVariant=Disabled  AWVariant=Passthrough  PCopyVariant=Disabled  TRVariant=Disabled  FdbkBlocksVariant=Forward  IdealPFdbkVariant=Disabled  SatFdbkVariant=Disabled  DerivativeFilterVariant=Disabled  NVariant=Disabled  NCopyVariant=Disabled_SignalSpec  FilterICVariant=Disabled  IntegratorICVariant=InternalICs  ExternalResetVariant=Disabled  TRSumVariant=Passthrough  SumFdbkVariant=Disabled  SumVariant=Sum_PI  TsampFilterVariant=InternalTs  TsampNgainVariant=Passthrough  TsampIntegralVariant=Disabled_SignalSpec  ExternalSaturationOutDataTypeStr=Inherit: Same as second input  DerivativeSourceVariant=Disabled  PreIntVariant=InternalPreInt
      settings: LibrarySourceBlock=simulink/Discrete/Discrete PID Controller
  Gain1 : Gain  Gain=1/0.01/0.005
  Gain2 : Gain  Gain=1/2
  Gain4 : Gain  Gain=P_base(6)/1e3
  Product{,1..5} (6 alike) : Product
  Saturation : Saturate  UpperLimit=1  LowerLimit=0.5
  Saturation1 : Saturate  UpperLimit=1  LowerLimit=0
  Scope1 : Scope  NumInputPorts=3
  Scope2 : Scope  NumInputPorts=2
  Step : Step  Time=15  SampleTime=0
  Sum : Sum  Inputs=|+-
  Sum1 : Sum  Inputs=|+-
  Sum2 : Sum  Inputs=|+-
  Sum3 : Sum  Inputs=|++
  Zero-Order Hold : ZeroOrderHold  SampleTime=ts_pi
  delta : Outport
  tag scope: delta_sapc6=global
  wires:
  Product/1 -> [delta_sapc6], Scope1/3, Discrete PID Controller/1
  Step/1 -> Product/2
  Sum/1 -> Gain4/1
  Discrete PID Controller/1 -> Scope1/1, Zero-Order Hold/1
  In1/1 -> Sum/1
  In2/1 -> Sum/2
  Zero-Order Hold/1 -> Scope1/2, delta/1
  Constant1/1 -> Product2/2
  Constant/1 -> Product1/1
  Product2/1 -> Scope2/2, Discrete PID Controller/3
  Product1/1 -> Scope2/1, Discrete PID Controller/2
  Saturation/1 -> Product2/1, Product1/2
  Constant4/1 -> Sum1/1
  Abs1/1 -> Product5/2, Sum1/2
  Constant3/1 -> Sum2/1
  Product3/1 -> Gain1/1
  Gain1/1 -> Sum2/2
  Gain4/1 -> Abs1/1, Product/1
  Sum2/1 -> Product4/2
  Product5/1 -> Saturation1/1
  Sum1/1 -> Product3/1, Product3/2
  Constant2/1 -> Product5/1
  Saturation1/1 -> Product4/1
  Delay2/1 -> Sum3/1
  Product4/1 -> Sum3/2, Delay2/1
  Gain2/1 -> Saturation/1
  Sum3/1 -> Gain2/1

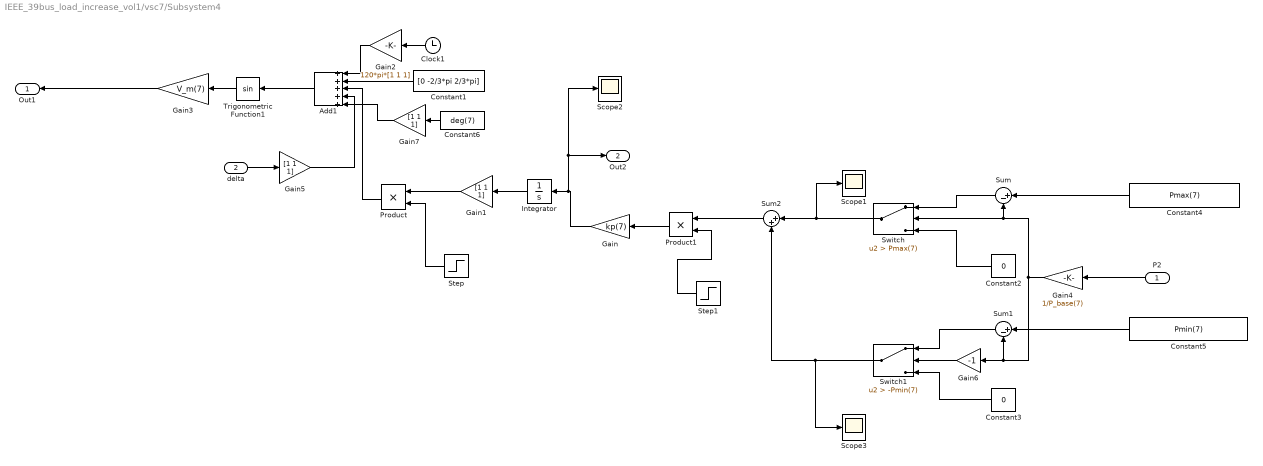
== system IEEE_39bus_load_increase_vol1/vsc7/Subsystem4 ==
  P2 : Inport
  delta : Inport  Port=2
  Add1 : Sum  Inputs=+++++
  Clock1 : Clock
  Constant1 : Constant  Value="[0  -2/3*pi   2/3*pi]"
  Constant2 : Constant  Value=0
  Constant3 : Constant  Value=0
  Constant4 : Constant  Value=Pmax(7)
  Constant5 : Constant  Value=Pmin(7)
  Constant6 : Constant  Value=deg(7)
  Gain : Gain  Gain=kp(7)
  Gain1 : Gain  Gain=[1 1 1]
  Gain2 : Gain  Gain=120*pi*[1 1 1]
  Gain3 : Gain  Gain=V_m(7)
  Gain4 : Gain  Gain=1/P_base(7)
  Gain5 : Gain  Gain=[1 1 1]
  Gain6 : Gain  Gain=-1
  Gain7 : Gain  Gain=[1 1 1]
  Integrator : Integrator
  Product : Product
  Product1 : Product
  Scope1 : Scope
  Scope2 : Scope
  Scope3 : Scope
  Step : Step  Time=5  SampleTime=0
  Step1 : Step  Time=5  SampleTime=0
  Sum : Sum  Inputs=|+-
  Sum1 : Sum  Inputs=|+-
  Sum2 : Sum  Inputs=|++
  Switch : Switch  Criteria=u2 > Threshold  Threshold=Pmax(7)  SaturateOnIntegerOverflow=off  InputSameDT=off
  Switch1 : Switch  Criteria=u2 > Threshold  Threshold=-Pmin(7)  SaturateOnIntegerOverflow=off  InputSameDT=off
  Trigonometric Function1 : Trigonometry
  Out1 : Outport
  Out2 : Outport  Port=2
  wires:
  Clock1/1 -> Gain2/1
  Constant1/1 -> Add1/2
  Gain2/1 -> Add1/1
  Add1/1 -> Trigonometric Function1/1
  Gain1/1 -> Product/1
  Step/1 -> Product/2
  Product/1 -> Add1/3
  Trigonometric Function1/1 -> Gain3/1
  Gain3/1 -> Out1/1
  P2/1 -> Gain4/1
  delta/1 -> Gain5/1
  Gain5/1 -> Add1/4
  Step1/1 -> Product1/2
  Constant4/1 -> Sum/1
  Sum/1 -> Switch/1
  Constant2/1 -> Switch/3
  Constant5/1 -> Sum1/1
  Sum1/1 -> Switch1/1
  Gain4/1 -> Gain6/1, Sum1/2, Sum/2, Switch/2
  Constant3/1 -> Switch1/3
  Gain6/1 -> Switch1/2
  Switch/1 -> Scope1/1, Sum2/1
  Switch1/1 -> Scope3/1, Sum2/2
  Sum2/1 -> Product1/1
  Constant6/1 -> Gain7/1
  Gain7/1 -> Add1/5
  Product1/1 -> Gain/1
  Integrator/1 -> Gain1/1
  Gain/1 -> Scope2/1, Out2/1, Integrator/1

== system IEEE_39bus_load_increase_vol1/vsc7/sapc ==
  In1 : Inport
  In2 : Inport  Port=2
  Discrete PID Controller : slpidlib/PID Controller  Controller=PI  Form=Parallel  TimeDomain=Discrete-time  UseExternalTs=off  SampleTime=-1  IntegratorMethod=Forward Euler  FilterMethod=Forward Euler  ControllerParametersSource=internal  P=kp_sapc*0.5  I=ki_sapc*0.2  UseKiTs=off  D=0  UseExternalDerivativeSource=off  N=100  UseFilter=on  TunerSelectOption=Transfer Function Based (PID Tuner App)  InitialConditionSource=internal  InitialConditionForIntegrator=0  InitialConditionForFilter=0  DifferentiatorICPrevScaledInput=0  ExternalReset=none  TrackingMode=off  Kt=1  LimitOutput=off  SatLimitsSource=internal  UpperSaturationLimit=inf  LowerSaturationLimit=-inf  LinearizeAsGain=off  AntiWindupMode=none  Kb=1  LimitIntegrator=off  UpperIntegratorSaturationLimit=inf  LowerIntegratorSaturationLimit=-inf  POutMin=[]  POutMax=[]  IOutMin=[]  IOutMax=[]  DOutMin=[]  DOutMax=[]  NOutMin=[]  NOutMax=[]  SumOutMin=[]  SumOutMax=[]  SaturationOutMin=[]  SaturationOutMax=[]  PParamMin=[]  PParamMax=[]  IParamMin=[]  IParamMax=[]  DParamMin=[]  DParamMax=[]  NParamMin=[]  NParamMax=[]  KbParamMin=[]  KbParamMax=[]  KtParamMin=[]  KtParamMax=[]  KbOutMin=[]  KbOutMax=[]  KtOutMin=[]  KtOutMax=[]  IntegratorOutMin=[]  IntegratorOutMax=[]  FilterOutMin=[]  FilterOutMax=[]  SumI1OutMin=[]  SumI1OutMax=[]  SumI2OutMin=[]  SumI2OutMax=[]  SumI3OutMin=[]  SumI3OutMax=[]  SumI4OutMin=[]  SumI4OutMax=[]  SumDOutMin=[]  SumDOutMax=[]  DifferentiatorOutMin=[]  DifferentiatorOutMax=[]  FilterDiffOutCoefMin=[]  FilterDiffOutCoefMax=[]  ReciprocalOutMin=[]  ReciprocalOutMax=[]  SumDenOutMin=[]  SumDenOutMax=[]  SumNumOutMin=[]  SumNumOutMax=[]  DivideOutMin=[]  DivideOutMax=[]  UdiffTsProdOutMin=[]  UdiffTsProdOutMax=[]  NTsProdOutMin=[]  NTsProdOutMax=[]  UintegralTsProdOutMin=[]  UintegralTsProdOutMax=[]  UngainTsProdOutMin=[]  UngainTsProdOutMax=[]  ClampingZeroOutDataTypeStr=Inherit: Inherit via back propagation  ClampingZeroOutMin=[]  ClampingZeroOutMax=[]  FilterDenConstantOutDataTypeStr=Inherit: Inherit via back propagation  FilterDenConstantOutMin=[]  FilterDenConstantOutMax=[]  PCopyOutDataTypeStr=Inherit: Inherit via back propagation  PCopyOutMin=[]  PCopyOutMax=[]  NCopyOutDataTypeStr=Inherit: Inherit via back propagation  NCopyOutMin=[]  NCopyOutMax=[]  IntegratorContinuousStateAttributes=''  IntegratorStateMustResolveToSignalObject=off  IntegratorRTWStateStorageClass=Auto  FilterContinuousStateAttributes=''  FilterStateMustResolveToSignalObject=off  FilterRTWStateStorageClass=Auto  ParallelPVariant=InternalParameters  IdealPVariant=Disabled  IVariant=InternalParameters  DVariant=Disabled  IntegratorVariant=Discrete  SatVariant=Disabled  AWVariant=Passthrough  PCopyVariant=Disabled  TRVariant=Disabled  FdbkBlocksVariant=Forward  IdealPFdbkVariant=Disabled  SatFdbkVariant=Disabled  DerivativeFilterVariant=Disabled  NVariant=Disabled  NCopyVariant=Disabled_SignalSpec  FilterICVariant=Disabled  IntegratorICVariant=InternalICs  ExternalResetVariant=Disabled  TRSumVariant=Passthrough  SumFdbkVariant=Disabled  SumVariant=Sum_PI  TsampFilterVariant=InternalTs  TsampNgainVariant=Passthrough  TsampIntegralVariant=Disabled_SignalSpec  ExternalSaturationOutDataTypeStr=Inherit: Same as second input  DerivativeSourceVariant=Disabled  PreIntVariant=InternalPreInt
      settings: LibrarySourceBlock=simulink/Discrete/Discrete PID Controller
  Gain4 : Gain  Gain=P_base(7)/1e3
  Goto10 : Goto  Commented=on  GotoTag=delta_sapc7  TagVisibility=global
  Product : Product
  Scope1 : Scope  NumInputPorts=2
  Step : Step  Time=15  SampleTime=0
  Sum : Sum  Inputs=|+-
  Zero-Order Hold : ZeroOrderHold  SampleTime=ts_pi
  delta : Outport
  wires:
  Product/1 -> Goto10/1, Scope1/2, Discrete PID Controller/1
  Step/1 -> Product/2
  Sum/1 -> Gain4/1
  Discrete PID Controller/1 -> Zero-Order Hold/1, Scope1/1
  In1/1 -> Sum/1
  In2/1 -> Sum/2
  Zero-Order Hold/1 -> delta/1
  Gain4/1 -> Product/1

== system IEEE_39bus_load_increase_vol1/vsc7/sapc1 ==
  In1 : Inport
  In2 : Inport  Port=2
  Abs1 : Abs  SaturateOnIntegerOverflow=off
  Constant : Constant  Value=kp_sapc
  Constant1 : Constant  Value=ki_sapc
  Constant2 : Constant  Value=1/0.015
  Constant3 : Constant
  Constant4 : Constant  Value=0.02
  Delay2 : Delay  DelayLength=1  InitialCondition=0  SampleTime=1e-4
  Discrete PID Controller : slpidlib/PID Controller  Controller=PI  Form=Parallel  TimeDomain=Discrete-time  UseExternalTs=off  SampleTime=-1  IntegratorMethod=Forward Euler  FilterMethod=Forward Euler  ControllerParametersSource=external  P=kp_sapc*2  I=ki_sapc*2  UseKiTs=off  D=0  UseExternalDerivativeSource=off  N=100  UseFilter=on  TunerSelectOption=Transfer Function Based (PID Tuner App)  InitialConditionSource=internal  InitialConditionForIntegrator=0  InitialConditionForFilter=0  DifferentiatorICPrevScaledInput=0  ExternalReset=none  TrackingMode=off  Kt=1  LimitOutput=off  SatLimitsSource=internal  UpperSaturationLimit=inf  LowerSaturationLimit=-inf  LinearizeAsGain=off  AntiWindupMode=none  Kb=1  LimitIntegrator=off  UpperIntegratorSaturationLimit=inf  LowerIntegratorSaturationLimit=-inf  POutMin=[]  POutMax=[]  IOutMin=[]  IOutMax=[]  DOutMin=[]  DOutMax=[]  NOutMin=[]  NOutMax=[]  SumOutMin=[]  SumOutMax=[]  SaturationOutMin=[]  SaturationOutMax=[]  PParamMin=[]  PParamMax=[]  IParamMin=[]  IParamMax=[]  DParamMin=[]  DParamMax=[]  NParamMin=[]  NParamMax=[]  KbParamMin=[]  KbParamMax=[]  KtParamMin=[]  KtParamMax=[]  KbOutMin=[]  KbOutMax=[]  KtOutMin=[]  KtOutMax=[]  IntegratorOutMin=[]  IntegratorOutMax=[]  FilterOutMin=[]  FilterOutMax=[]  SumI1OutMin=[]  SumI1OutMax=[]  SumI2OutMin=[]  SumI2OutMax=[]  SumI3OutMin=[]  SumI3OutMax=[]  SumI4OutMin=[]  SumI4OutMax=[]  SumDOutMin=[]  SumDOutMax=[]  DifferentiatorOutMin=[]  DifferentiatorOutMax=[]  FilterDiffOutCoefMin=[]  FilterDiffOutCoefMax=[]  ReciprocalOutMin=[]  ReciprocalOutMax=[]  SumDenOutMin=[]  SumDenOutMax=[]  SumNumOutMin=[]  SumNumOutMax=[]  DivideOutMin=[]  DivideOutMax=[]  UdiffTsProdOutMin=[]  UdiffTsProdOutMax=[]  NTsProdOutMin=[]  NTsProdOutMax=[]  UintegralTsProdOutMin=[]  UintegralTsProdOutMax=[]  UngainTsProdOutMin=[]  UngainTsProdOutMax=[]  ClampingZeroOutDataTypeStr=Inherit: Inherit via back propagation  ClampingZeroOutMin=[]  ClampingZeroOutMax=[]  FilterDenConstantOutDataTypeStr=Inherit: Inherit via back propagation  FilterDenConstantOutMin=[]  FilterDenConstantOutMax=[]  PCopyOutDataTypeStr=Inherit: Inherit via back propagation  PCopyOutMin=[]  PCopyOutMax=[]  NCopyOutDataTypeStr=Inherit: Inherit via back propagation  NCopyOutMin=[]  NCopyOutMax=[]  IntegratorContinuousStateAttributes=''  IntegratorStateMustResolveToSignalObject=off  IntegratorRTWStateStorageClass=Auto  FilterContinuousStateAttributes=''  FilterStateMustResolveToSignalObject=off  FilterRTWStateStorageClass=Auto  ParallelPVariant=ExternalParameters  IdealPVariant=Disabled  IVariant=ExternalParameters  DVariant=Disabled  IntegratorVariant=Discrete  SatVariant=Disabled  AWVariant=Passthrough  PCopyVariant=Disabled  TRVariant=Disabled  FdbkBlocksVariant=Forward  IdealPFdbkVariant=Disabled  SatFdbkVariant=Disabled  DerivativeFilterVariant=Disabled  NVariant=Disabled  NCopyVariant=Disabled_SignalSpec  FilterICVariant=Disabled  IntegratorICVariant=InternalICs  ExternalResetVariant=Disabled  TRSumVariant=Passthrough  SumFdbkVariant=Disabled  SumVariant=Sum_PI  TsampFilterVariant=InternalTs  TsampNgainVariant=Passthrough  TsampIntegralVariant=Disabled_SignalSpec  ExternalSaturationOutDataTypeStr=Inherit: Same as second input  DerivativeSourceVariant=Disabled  PreIntVariant=InternalPreInt
      settings: LibrarySourceBlock=simulink/Discrete/Discrete PID Controller
  Gain1 : Gain  Gain=1/0.01/0.005
  Gain2 : Gain  Gain=1/2
  Gain4 : Gain  Gain=P_base(7)/1e3
  Product{,1..5} (6 alike) : Product
  Saturation : Saturate  UpperLimit=1  LowerLimit=0.5
  Saturation1 : Saturate  UpperLimit=1  LowerLimit=0
  Scope1 : Scope  NumInputPorts=3
  Scope2 : Scope  NumInputPorts=2
  Step : Step  Time=15  SampleTime=0
  Sum : Sum  Inputs=|+-
  Sum1 : Sum  Inputs=|+-
  Sum2 : Sum  Inputs=|+-
  Sum3 : Sum  Inputs=|++
  Zero-Order Hold : ZeroOrderHold  SampleTime=ts_pi
  delta : Outport
  tag scope: delta_sapc7=global
  wires:
  Product/1 -> [delta_sapc7], Scope1/3, Discrete PID Controller/1
  Step/1 -> Product/2
  Sum/1 -> Gain4/1
  Discrete PID Controller/1 -> Scope1/1, Zero-Order Hold/1
  In1/1 -> Sum/1
  In2/1 -> Sum/2
  Zero-Order Hold/1 -> Scope1/2, delta/1
  Constant1/1 -> Product2/2
  Constant/1 -> Product1/1
  Product2/1 -> Scope2/2, Discrete PID Controller/3
  Product1/1 -> Scope2/1, Discrete PID Controller/2
  Saturation/1 -> Product2/1, Product1/2
  Constant4/1 -> Sum1/1
  Abs1/1 -> Product5/2, Sum1/2
  Constant3/1 -> Sum2/1
  Product3/1 -> Gain1/1
  Gain1/1 -> Sum2/2
  Gain4/1 -> Abs1/1, Product/1
  Sum2/1 -> Product4/2
  Product5/1 -> Saturation1/1
  Sum1/1 -> Product3/1, Product3/2
  Constant2/1 -> Product5/1
  Saturation1/1 -> Product4/1
  Delay2/1 -> Sum3/1
  Product4/1 -> Sum3/2, Delay2/1
  Gain2/1 -> Saturation/1
  Sum3/1 -> Gain2/1

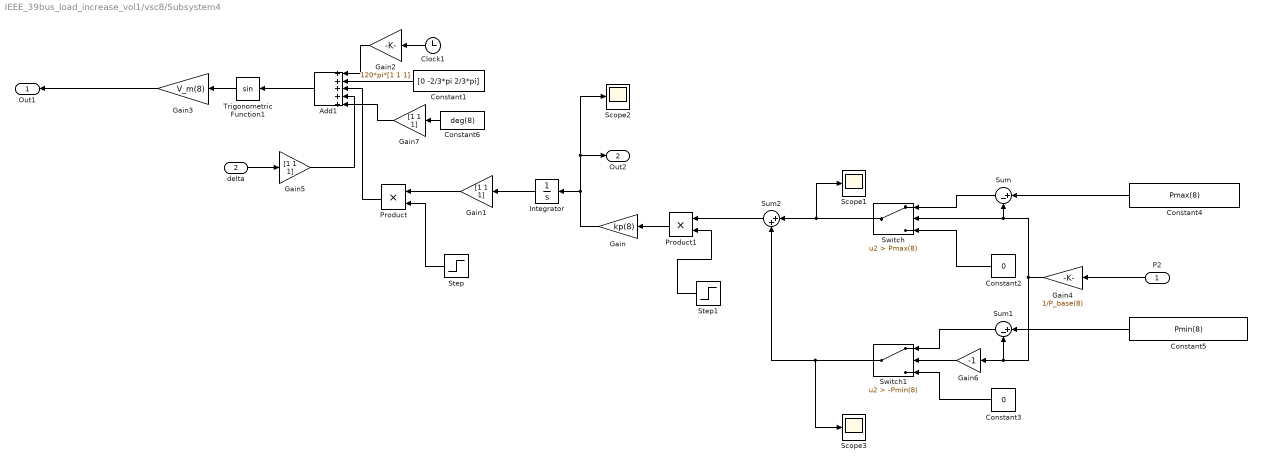
== system IEEE_39bus_load_increase_vol1/vsc8/Subsystem4 ==
  P2 : Inport
  delta : Inport  Port=2
  Add1 : Sum  Inputs=+++++
  Clock1 : Clock
  Constant1 : Constant  Value="[0  -2/3*pi   2/3*pi]"
  Constant2 : Constant  Value=0
  Constant3 : Constant  Value=0
  Constant4 : Constant  Value=Pmax(8)
  Constant5 : Constant  Value=Pmin(8)
  Constant6 : Constant  Value=deg(8)
  Gain : Gain  Gain=kp(8)
  Gain1 : Gain  Gain=[1 1 1]
  Gain2 : Gain  Gain=120*pi*[1 1 1]
  Gain3 : Gain  Gain=V_m(8)
  Gain4 : Gain  Gain=1/P_base(8)
  Gain5 : Gain  Gain=[1 1 1]
  Gain6 : Gain  Gain=-1
  Gain7 : Gain  Gain=[1 1 1]
  Integrator : Integrator
  Product : Product
  Product1 : Product
  Scope1 : Scope
  Scope2 : Scope
  Scope3 : Scope
  Step : Step  Time=5  SampleTime=0
  Step1 : Step  Time=5  SampleTime=0
  Sum : Sum  Inputs=|+-
  Sum1 : Sum  Inputs=|+-
  Sum2 : Sum  Inputs=|++
  Switch : Switch  Criteria=u2 > Threshold  Threshold=Pmax(8)  SaturateOnIntegerOverflow=off  InputSameDT=off
  Switch1 : Switch  Criteria=u2 > Threshold  Threshold=-Pmin(8)  SaturateOnIntegerOverflow=off  InputSameDT=off
  Trigonometric Function1 : Trigonometry
  Out1 : Outport
  Out2 : Outport  Port=2
  wires:
  Clock1/1 -> Gain2/1
  Constant1/1 -> Add1/2
  Gain2/1 -> Add1/1
  Add1/1 -> Trigonometric Function1/1
  Gain1/1 -> Product/1
  Step/1 -> Product/2
  Product/1 -> Add1/3
  Trigonometric Function1/1 -> Gain3/1
  Gain3/1 -> Out1/1
  P2/1 -> Gain4/1
  delta/1 -> Gain5/1
  Gain5/1 -> Add1/4
  Step1/1 -> Product1/2
  Constant4/1 -> Sum/1
  Sum/1 -> Switch/1
  Constant2/1 -> Switch/3
  Constant5/1 -> Sum1/1
  Sum1/1 -> Switch1/1
  Gain4/1 -> Gain6/1, Sum1/2, Sum/2, Switch/2
  Constant3/1 -> Switch1/3
  Gain6/1 -> Switch1/2
  Switch/1 -> Scope1/1, Sum2/1
  Switch1/1 -> Scope3/1, Sum2/2
  Sum2/1 -> Product1/1
  Constant6/1 -> Gain7/1
  Gain7/1 -> Add1/5
  Integrator/1 -> Gain1/1
  Gain/1 -> Scope2/1, Out2/1, Integrator/1
  Product1/1 -> Gain/1

== system IEEE_39bus_load_increase_vol1/vsc8/sapc ==
  In1 : Inport
  In2 : Inport  Port=2
  Discrete PID Controller : slpidlib/PID Controller  Controller=PI  Form=Parallel  TimeDomain=Discrete-time  UseExternalTs=off  SampleTime=-1  IntegratorMethod=Forward Euler  FilterMethod=Forward Euler  ControllerParametersSource=internal  P=kp_sapc  I=ki_sapc  UseKiTs=off  D=0  UseExternalDerivativeSource=off  N=100  UseFilter=on  TunerSelectOption=Transfer Function Based (PID Tuner App)  InitialConditionSource=internal  InitialConditionForIntegrator=0  InitialConditionForFilter=0  DifferentiatorICPrevScaledInput=0  ExternalReset=none  TrackingMode=off  Kt=1  LimitOutput=off  SatLimitsSource=internal  UpperSaturationLimit=inf  LowerSaturationLimit=-inf  LinearizeAsGain=off  AntiWindupMode=none  Kb=1  LimitIntegrator=off  UpperIntegratorSaturationLimit=inf  LowerIntegratorSaturationLimit=-inf  POutMin=[]  POutMax=[]  IOutMin=[]  IOutMax=[]  DOutMin=[]  DOutMax=[]  NOutMin=[]  NOutMax=[]  SumOutMin=[]  SumOutMax=[]  SaturationOutMin=[]  SaturationOutMax=[]  PParamMin=[]  PParamMax=[]  IParamMin=[]  IParamMax=[]  DParamMin=[]  DParamMax=[]  NParamMin=[]  NParamMax=[]  KbParamMin=[]  KbParamMax=[]  KtParamMin=[]  KtParamMax=[]  KbOutMin=[]  KbOutMax=[]  KtOutMin=[]  KtOutMax=[]  IntegratorOutMin=[]  IntegratorOutMax=[]  FilterOutMin=[]  FilterOutMax=[]  SumI1OutMin=[]  SumI1OutMax=[]  SumI2OutMin=[]  SumI2OutMax=[]  SumI3OutMin=[]  SumI3OutMax=[]  SumI4OutMin=[]  SumI4OutMax=[]  SumDOutMin=[]  SumDOutMax=[]  DifferentiatorOutMin=[]  DifferentiatorOutMax=[]  FilterDiffOutCoefMin=[]  FilterDiffOutCoefMax=[]  ReciprocalOutMin=[]  ReciprocalOutMax=[]  SumDenOutMin=[]  SumDenOutMax=[]  SumNumOutMin=[]  SumNumOutMax=[]  DivideOutMin=[]  DivideOutMax=[]  UdiffTsProdOutMin=[]  UdiffTsProdOutMax=[]  NTsProdOutMin=[]  NTsProdOutMax=[]  UintegralTsProdOutMin=[]  UintegralTsProdOutMax=[]  UngainTsProdOutMin=[]  UngainTsProdOutMax=[]  ClampingZeroOutDataTypeStr=Inherit: Inherit via back propagation  ClampingZeroOutMin=[]  ClampingZeroOutMax=[]  FilterDenConstantOutDataTypeStr=Inherit: Inherit via back propagation  FilterDenConstantOutMin=[]  FilterDenConstantOutMax=[]  PCopyOutDataTypeStr=Inherit: Inherit via back propagation  PCopyOutMin=[]  PCopyOutMax=[]  NCopyOutDataTypeStr=Inherit: Inherit via back propagation  NCopyOutMin=[]  NCopyOutMax=[]  IntegratorContinuousStateAttributes=''  IntegratorStateMustResolveToSignalObject=off  IntegratorRTWStateStorageClass=Auto  FilterContinuousStateAttributes=''  FilterStateMustResolveToSignalObject=off  FilterRTWStateStorageClass=Auto  ParallelPVariant=InternalParameters  IdealPVariant=Disabled  IVariant=InternalParameters  DVariant=Disabled  IntegratorVariant=Discrete  SatVariant=Disabled  AWVariant=Passthrough  PCopyVariant=Disabled  TRVariant=Disabled  FdbkBlocksVariant=Forward  IdealPFdbkVariant=Disabled  SatFdbkVariant=Disabled  DerivativeFilterVariant=Disabled  NVariant=Disabled  NCopyVariant=Disabled_SignalSpec  FilterICVariant=Disabled  IntegratorICVariant=InternalICs  ExternalResetVariant=Disabled  TRSumVariant=Passthrough  SumFdbkVariant=Disabled  SumVariant=Sum_PI  TsampFilterVariant=InternalTs  TsampNgainVariant=Passthrough  TsampIntegralVariant=Disabled_SignalSpec  ExternalSaturationOutDataTypeStr=Inherit: Same as second input  DerivativeSourceVariant=Disabled  PreIntVariant=InternalPreInt
      settings: LibrarySourceBlock=simulink/Discrete/Discrete PID Controller
  Gain4 : Gain  Gain=P_base(8)/1e3
  Product : Product
  Scope1 : Scope  NumInputPorts=2
  Step : Step  Time=15  SampleTime=0
  Sum : Sum  Inputs=|+-
  Zero-Order Hold : ZeroOrderHold  SampleTime=ts_pi
  delta : Outport
  wires:
  Product/1 -> Scope1/2, Discrete PID Controller/1
  Step/1 -> Product/2
  Sum/1 -> Gain4/1
  Discrete PID Controller/1 -> Zero-Order Hold/1, Scope1/1
  In1/1 -> Sum/1
  In2/1 -> Sum/2
  Zero-Order Hold/1 -> delta/1
  Gain4/1 -> Product/1
